simulink library "snellLeastSquaresPosition_ul"  (R2018b)
settings: Solver=VariableStepAuto  StartTime=0.0  StopTime=10.0  RelTol=1e-3
settings Model: Creator=MAE-NCSUCORE  LastModifiedBy=MAE-NCSUCORE

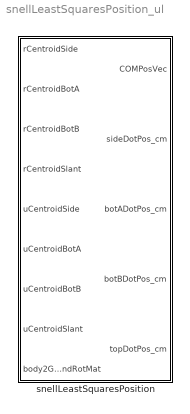
== system snellLeastSquaresPosition_ul ==
  snellLeastSquaresPosition : Subsystem  mask{sideDotPosVec_cm=0, botADotPosVec_cm=0, botBDotPosVec_cm=0, topDotPosVec_cm=0}
      mask prompts: sideDotPosVec_cm "Side Dot Position Vector [cm]"; botADotPosVec_cm "Bottom Dot A Position Vector [cm]"; botBDotPosVec_cm "Bottom Dot B Position Vector [cm]"; topDotPosVec_cm "Top Dot Position Vector [cm]"

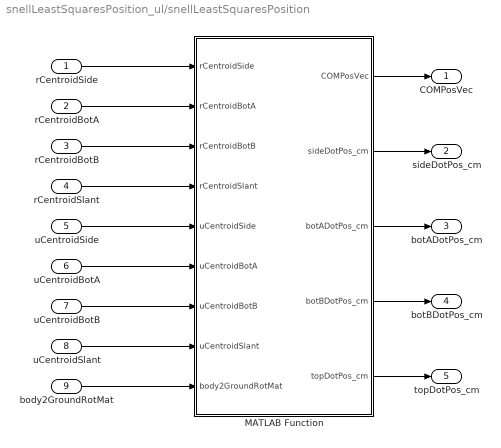
== system snellLeastSquaresPosition_ul/snellLeastSquaresPosition ==
  rCentroidSide : Inport
  rCentroidBotA : Inport  Port=2
  rCentroidBotB : Inport  Port=3
  rCentroidSlant : Inport  Port=4
  uCentroidSide : Inport  Port=5
  uCentroidBotA : Inport  Port=6
  uCentroidBotB : Inport  Port=7
  uCentroidSlant : Inport  Port=8
  body2GroundRotMat : Inport  Port=9
  MATLAB Function : MATLAB Function  TreatAsAtomicUnit=on
  COMPosVec : Outport
  sideDotPos_cm : Outport  Port=2
  botADotPos_cm : Outport  Port=3
  botBDotPos_cm : Outport  Port=4
  topDotPos_cm : Outport  Port=5
  wires:
  body2GroundRotMat/1 -> MATLAB Function/9(body2GroundRotMat)
  MATLAB Function/1(COMPosVec) -> COMPosVec/1
  uCentroidSlant/1 -> MATLAB Function/8(uCentroidSlant)
  uCentroidBotB/1 -> MATLAB Function/7(uCentroidBotB)
  uCentroidBotA/1 -> MATLAB Function/6(uCentroidBotA)
  uCentroidSide/1 -> MATLAB Function/5(uCentroidSide)
  rCentroidSlant/1 -> MATLAB Function/4(rCentroidSlant)
  rCentroidBotB/1 -> MATLAB Function/3(rCentroidBotB)
  rCentroidBotA/1 -> MATLAB Function/2(rCentroidBotA)
  rCentroidSide/1 -> MATLAB Function/1(rCentroidSide)
  MATLAB Function/3(botADotPos_cm) -> botADotPos_cm/1
  MATLAB Function/2(sideDotPos_cm) -> sideDotPos_cm/1
  MATLAB Function/4(botBDotPos_cm) -> botBDotPos_cm/1
  MATLAB Function/5(topDotPos_cm) -> topDotPos_cm/1

== matlab function snellLeastSquaresPosition_ul/snellLeastSquaresPosition/MATLAB Function ==
  data: rCentroidSide input; COMPosVec output; rCentroidBotA input; rCentroidBotB input; rCentroidSlant input; uCentroidSide input; uCentroidBotA input; uCentroidBotB input; uCentroidSlant input; body2GroundRotMat input; sideDotPosVec_cm parameter; botADotPosVec_cm parameter; botBDotPosVec_cm parameter; sideDotPos_cm output; botADotPos_cm output; botBDotPos_cm output; topDotPos_cm output; topDotPosVec_cm parameter
function [COMPosVec,sideDotPos_cm,botADotPos_cm,botBDotPos_cm,topDotPos_cm]...
    = snellLeastSquaresPosition(...
    rCentroidSide,...
    rCentroidBotA,...
    rCentroidBotB,...
    rCentroidSlant,...
    uCentroidSide,...
    uCentroidBotA,...
    uCentroidBotB,...
    uCentroidSlant,...
    body2GroundRotMat,...
    sideDotPosVec_cm,botADotPosVec_cm,botBDotPosVec_cm,topDotPosVec_cm)

[COMPosVec,sideDotPos_cm,botADotPos_cm,botBDotPos_cm,topDotPos_cm]...
    = snellLeastSquaresPosition(...
    rCentroidSide,...
    rCentroidBotA,...
    rCentroidBotB,...
    rCentroidSlant,...
    uCentroidSide,...
    uCentroidBotA,...
    uCentroidBotB,...
    uCentroidSlant,...
    body2GroundRotMat,...
    sideDotPosVec_cm,botADotPosVec_cm,botBDotPosVec_cm,topDotPosVec_cm);
